simulink model "ClosedLoopSim"  (R2022b)
settings: Solver=ode15s  StartTime=0.0  StopTime=Tmax  RelTol=1e-3
values from neighbouring files (symbols this model uses):
  mod = mod.train(trainDat,4,0.95,0.95,false)    [main.m]
  pmod = mod.p    [main.m]
  r0 = 0.6    [main.m]
undefined symbols (not defined in the file or in its folder): sauter
libraries: mpclib x1
settings Model: Creator=IFAT  LastModifiedBy=eotto

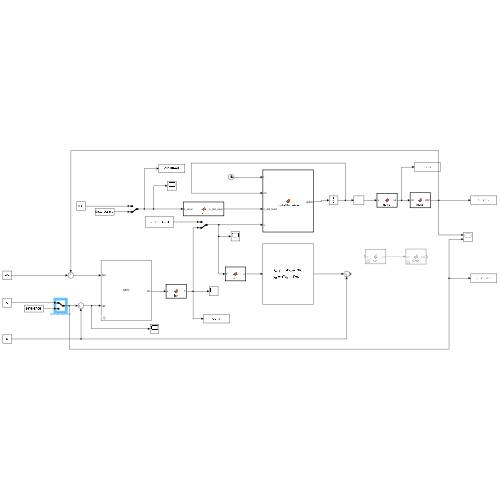
[thumbnail: Simulink's stored preview of the top-level diagram]
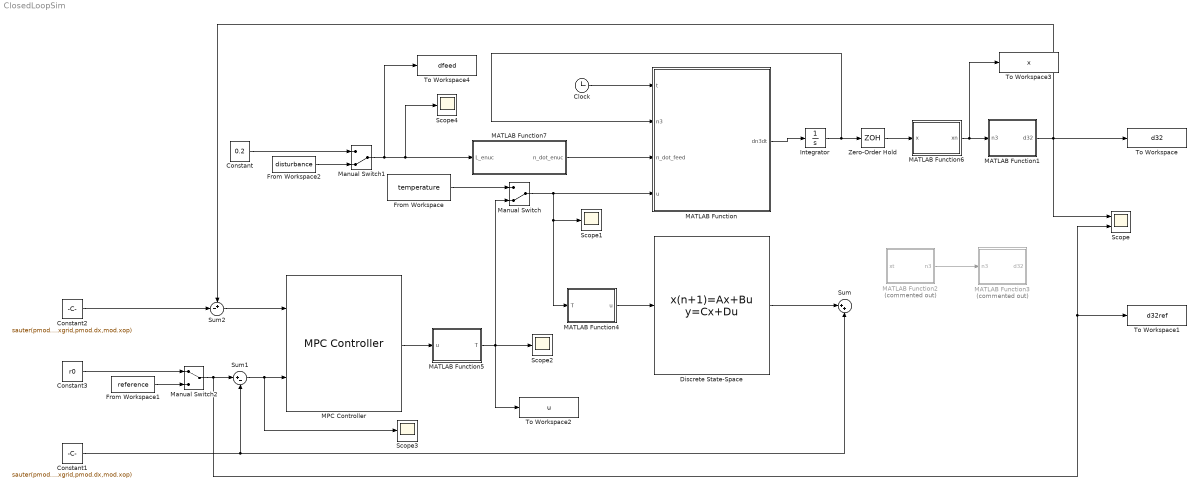
== system ClosedLoopSim ==
  Clock : Clock
  Constant : Constant  Value=0.2
  Constant1 : Constant  Value=sauter(pmod.xgrid,pmod.dx,mod.xop)
  Constant2 : Constant  Value=sauter(pmod.xgrid,pmod.dx,mod.xop)  SampleTime=0
  Constant3 : Constant  Value=r0
  Discrete State-Space : DiscreteStateSpace  A=mod.stateSpace.A  B=mod.stateSpace.B  C=mod.stateSpace.C  D=mod.stateSpace.D  SampleTime=mod.stateSpace.ts
  From Workspace : FromWorkspace  VariableName=temperature  SampleTime=1
  From Workspace1 : FromWorkspace  VariableName=reference
  From Workspace2 : FromWorkspace  VariableName=disturbance
  Integrator : Integrator  InitialCondition=mod.xop
  MATLAB Function : MATLAB Function  TreatAsAtomicUnit=on
  MATLAB Function1 : MATLAB Function  TreatAsAtomicUnit=on
  MATLAB Function2 : MATLAB Function  Commented=on  TreatAsAtomicUnit=on
  MATLAB Function3 : MATLAB Function  Commented=on  TreatAsAtomicUnit=on
  MATLAB Function4 : MATLAB Function  TreatAsAtomicUnit=on
  MATLAB Function5 : MATLAB Function  TreatAsAtomicUnit=on
  MATLAB Function6 : MATLAB Function  TreatAsAtomicUnit=on
  MATLAB Function7 : MATLAB Function  TreatAsAtomicUnit=on
  MPC Controller : mpclib/MPC Controller  SCDEnableBlockLinearizationSpecification=on  mpcobj=mpcobj  is_multiple=0  enable_value=0  return_u0=off  updateMPCinCallerWorkspace=on  md_inport=off  mv_inport=off  uref_inport=off  return_cost=off  return_mvseq=off  return_qpstatus=off  return_xseq=off  return_state=off  return_ovseq=off  state_inport=off  umin_inport=off  umax_inport=off  ymin_inport=off  ymax_inport=off  cc_inport=off  ywt_inport=off  uwt_inport=off  duwt_inport=off  rhoeps_inport=off  pm_inport=off  MaximumP=10  HorizonChoice=FixedHorizon  n_ts=60  n_p=30  n_mv=1  n_md=0  n_ud=0  n_mo=1  n_uo=0  BlockDataType=double  SampleTimeInherited=off  switch_inport=off
  Manual Switch : ManualSwitch  CurrentSetting=0
  Manual Switch1 : ManualSwitch  CurrentSetting=0
  Manual Switch2 : ManualSwitch
  Scope : Scope  NumInputPorts=2
  Scope{1..4} (4 alike) : Scope
  Sum : Sum  Inputs=|++
  Sum1 : Sum  Inputs=|+-
  Sum2 : Sum  Inputs=+-|
  To Workspace : ToWorkspace  VariableName=d32  SampleTime=mod.ts
  To Workspace1 : ToWorkspace  VariableName=d32ref  SampleTime=mod.ts
  To Workspace2 : ToWorkspace  VariableName=u  SampleTime=mod.ts
  To Workspace3 : ToWorkspace  VariableName=x  SampleTime=mod.ts
  To Workspace4 : ToWorkspace  VariableName=dfeed  SampleTime=mod.ts
  Zero-Order Hold : ZeroOrderHold  SampleTime=mod.ts
  wires:
  Clock/1 -> MATLAB Function/1(t)
  MATLAB Function/1(dn3dt) -> Integrator/1
  Integrator/1 -> Zero-Order Hold/1, MATLAB Function/2(n3)
  MATLAB Function4/1(u) -> Discrete State-Space/1
  MATLAB Function2/1(n3) -> MATLAB Function3/1(n3)
  Manual Switch/1 -> MATLAB Function4/1(T), Scope1/1, MATLAB Function/4(u)
  From Workspace/1 -> Manual Switch/1
  Discrete State-Space/1 -> Sum/1
  Constant1/1 -> Sum/2, Sum1/2
  Sum1/1 -> Scope3/1, MPC Controller/2
  MPC Controller/1 -> MATLAB Function5/1(u)
  MATLAB Function5/1(T) -> To Workspace2/1, Manual Switch/2, Scope2/1
  Constant2/1 -> Sum2/2
  Sum2/1 -> MPC Controller/1
  Zero-Order Hold/1 -> MATLAB Function6/1(x)
  MATLAB Function1/1(d32) -> To Workspace/1, Scope/1, Sum2/1
  MATLAB Function6/1(xn) -> To Workspace3/1, MATLAB Function1/1(n3)
  MATLAB Function7/1(n_dot_enuc) -> MATLAB Function/3(n_dot_feed)
  Manual Switch1/1 -> To Workspace4/1, Scope4/1, MATLAB Function7/1(L_enuc)
  From Workspace2/1 -> Manual Switch1/2
  Constant/1 -> Manual Switch1/1
  Manual Switch2/1 -> Scope/2, To Workspace1/1, Sum1/1
  From Workspace1/1 -> Manual Switch2/2
  Constant3/1 -> Manual Switch2/1

== matlab function ClosedLoopSim/MATLAB Function1 ==
  data: n3 input; d32 output; pmod parameter
function d32 = meas(n3, pmod)

    d32 = sauter(pmod.xgrid,pmod.dx,n3);

end

== matlab function ClosedLoopSim/MATLAB Function ==
  data: t input; n3 input; n_dot_feed input; u input; dn3dt output; pagg parameter
function dn3dt = nonlinSimulation(t,n3,n_dot_feed,u, pagg)
    p = pagg; 
    p.n_dot_enuc = n_dot_feed;
    dn3dt = proces(t,n3,p,@(t) u);
end

== matlab function ClosedLoopSim/MATLAB Function2 ==
  data: xt input; pmod parameter; n3 output size=[pagg.N,1]
function n3 = fcn(xt, pmod)

    x = pmod.U*xt;

    n3 = inverseCoordinateTransformation(pmod.N_x,pmod.N_x_transformed,pmod.N_del,...
                pmod.xop,pmod.stateScale,pmod.inputScale,pmod.ext,x);
end

== matlab function ClosedLoopSim/MATLAB Function3 ==
  data: n3 input; d32 output; pmod parameter
function d32 = meas(n3, pmod)

    d32 = sauter(pmod.xgrid,pmod.dx,n3);

end

== matlab function ClosedLoopSim/MATLAB Function4 ==
  data: T input; u output; pmod parameter
function u = fcn(T,pmod)
    u = (T - pmod.uop)/pmod.inputScale;
end

== matlab function ClosedLoopSim/MATLAB Function5 ==
  data: u input; T output; pmod parameter
function T = fcn(u,pmod)

T = u*pmod.inputScale + pmod.uop;

== matlab function ClosedLoopSim/MATLAB Function6 ==
  data: x input; xn output; pmod parameter
function xn = noise(x,pmod)

    xn = noise(x);

end

== matlab function ClosedLoopSim/MATLAB Function7 ==
  data: L_enuc input; n_dot_enuc output; pagg parameter
function n_dot_enuc = fcn(L_enuc, pagg)
    p = pagg;
    m_dot_enuc    =       0.25/60;    % [kg/s]
    sig_enuc      =       0.02;
    n_dot_enuc = generateFeed(m_dot_enuc,L_enuc,sig_enuc,p.xgrid,p.dx,p.dv,p.rho_p);
end
